simulink model "qcarLidarToGPS"  (R2021a)
settings: Solver=ode1  StartTime=0.0  StopTime=inf  FixedStep=1/15  RelTol=1e-3  EnableMultiTasking=on
undefined symbols (not defined in the file): qc_get_step_size
libraries: quarc_library x18, simulink x2
settings Model: SimulationMode=external  ExtModeTrigDuration=10000  Creator=PKaram  LastModifiedBy=mrushton
settings SolverCC: AlgebraicLoopSolver=TrustRegion  PositivePriorityOrder=on  AutoInsertRateTranBlk=on
settings DataIOCC: ReturnWorkspaceOutputs=off
settings DebuggingCC: ParameterPrecisionLossMsg=none  SFMachineParentedDataDiag=warning  ArithmeticOperatorsInVariantConditions=warning
settings HardwareCC: ProdBitPerLong=64  ProdLargestAtomicFloat=None  ProdEndianess=Unspecified  ProdHWDeviceType=Generic->64-bit Embedded Processor (LP64)
settings SFSimCC: SimUseLocalCustomCode=off  CustomCodeUndefinedFunction=UseInterfaceOnly
settings RTWCC: Description=QUARC Linux Nvidia Target (QCar) Using Toolchain  SystemTargetFile=quarc_linux_nvidia.tlc  TemplateMakefile=quarc_linux_nvidia_tmf  RTWUseLocalCustomCode=off  Toolchain=QUARC linux_nvidia | gmake (64-bit Windows)  BuildConfiguration=Faster Runs
settings CodeAppCC: StateflowObjectComments=on
settings STFCustomTargetCC: TargetLangStandard=C99 (ISO)  ConcurrentExecutionCompliant=on  SystemTargetFile=quarc_linux_nvidia.tlc
settings GRTTargetCC: ParMdlRefBuildCompliant=off  CompOptLevelCompliant=off  CombineOutputUpdateFcns=off  MatFileLogging=off  CPPClassGenCompliant=off  GRTInterface=on  ExtMode=on  ExtModeMexFile=quarc_comm  ExtModeMexArgs='-w -d /tmp -uri %u -pose_0 5.2,3.4,6.5','tcpip://192.168.55.1:17001'
settings ConfigComp: CovMetricSettings=dswe

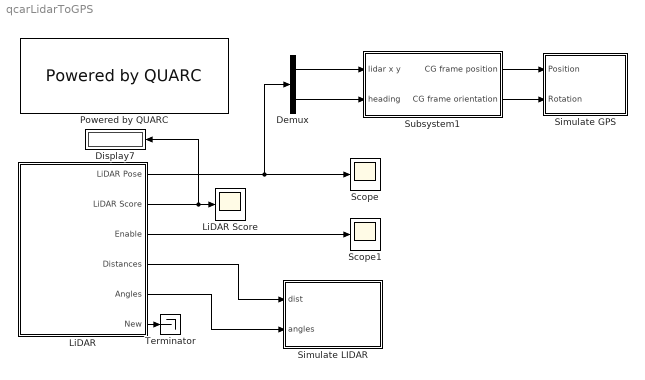
== system qcarLidarToGPS ==
  Demux : Demux  Outputs=[2 1]
  Display7 : Display
  LiDAR : Subsystem
  LiDAR Score : Scope
  Powered by QUARC : quarc_library/Logos/Powered by QUARC
  Scope : Scope
  Scope1 : Scope
  Simulate GPS : Subsystem
  Simulate LIDAR : Subsystem
  Subsystem1 : Subsystem
  Terminator : Terminator
  wires:
  LiDAR/2("LiDAR Score ") -> Display7/1, LiDAR Score/1
  LiDAR/3(Enable) -> Scope1/1
  LiDAR/1(LiDAR Pose) -> Scope/1, Demux/1
  Demux/1 -> Subsystem1/1(lidar x y)
  Subsystem1/1("CG frame position ") -> Simulate GPS/1(Position)
  Subsystem1/2(CG frame orientation) -> Simulate GPS/2(Rotation)
  Demux/2 -> Subsystem1/2(heading)
  LiDAR/4(Distances) -> Simulate LIDAR/1(dist)
  LiDAR/5(Angles) -> Simulate LIDAR/2(angles)
  LiDAR/6(New) -> Terminator/1

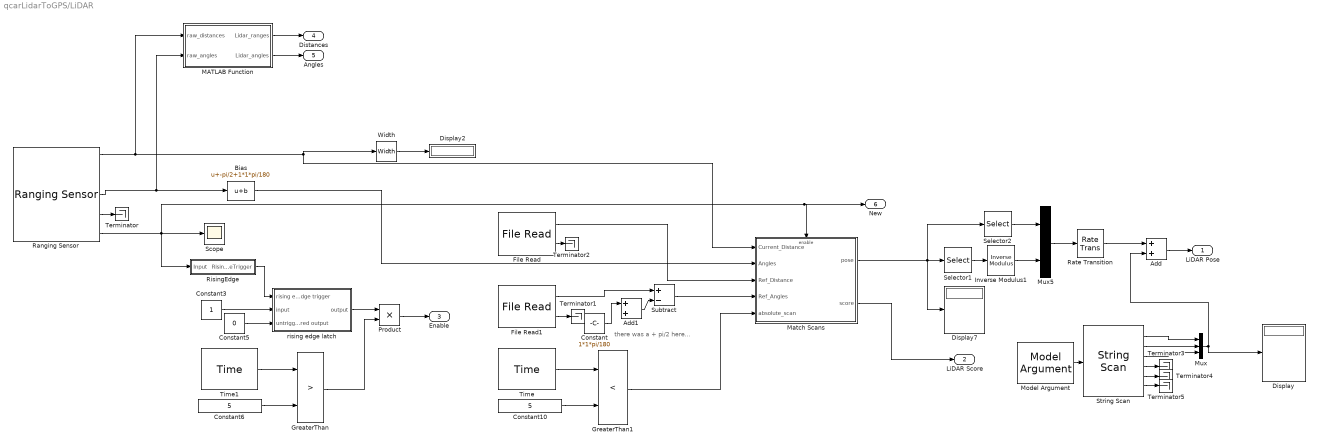
== system qcarLidarToGPS/LiDAR ==
  note: there was a + pi/2 here...
  Add : Sum
  Add1 : Sum
  Bias : Bias  Bias=-pi/2+1*1*pi/180
  Constant : Constant  Value=1*1*pi/180
  Constant10 : Constant  Value=5
  Constant3 : Constant
  Constant5 : Constant  Value=0
  Constant6 : Constant  Value=5
  Display : Display
  Display2 : Display
  Display7 : Display
  File Read : quarc_library/Sources/Signals/File Read  filename=distance_new.mat  format=MAT-file v.4  variable=distances  dimensions=[384, 1]  skip_lines=1  skip_columns=1  loop_count=0  sample_time=qc_get_step_size  data_type=double
      settings: AttributesFormatString=%<filename>  SourceProductName=QUARC Targets
  File Read1 : quarc_library/Sources/Signals/File Read  filename=angles_new.mat  format=MAT-file v.4  variable=angles  dimensions=[384, 1]  skip_lines=1  skip_columns=1  loop_count=0  sample_time=qc_get_step_size  data_type=double
      settings: AttributesFormatString=%<filename>  SourceProductName=QUARC Targets
  GreaterThan : RelationalOperator  Operator=>  OutDataTypeStr=boolean  RndMeth=Simplest
  GreaterThan1 : RelationalOperator  Operator=<  OutDataTypeStr=boolean  RndMeth=Simplest
  Inverse Modulus1 : quarc_library/Discontinuities/Inverse Modulus  modulus=2*pi  output_derivative=off  output_revolutions=off  max_x=Inf  min_x=-Inf
  MATLAB Function : MATLAB Function  TreatAsAtomicUnit=on
  Match Scans : Subsystem
  Model Argument : quarc_library/Sources/Signals/Model Argument  argument_name=pose_0  has_value=on  data_type_mode=Specify via dialog  data_type=char  max_length=80  default_value=0  variable_size=on
      settings: AttributesFormatString=(-%<argument_name>)  SourceProductName=QUARC Targets
  Mux : Mux  Inputs=3
  Mux5 : Mux  Inputs=2
  Product : Product
  Ranging Sensor : quarc_library/Devices/Third-Party/Sensors/Ranging Sensor  sensor_type=RPLidar LIDAR  uri=serial-cpu://localhost:2?baud='115200',word='8',parity='none',stop='1',flow='none',dsr='on'  ranging_distance=Long  timing_budget=0.033  measurement_period=0.040  output_mode=Variable-size output  samples_per_revolution=384  max_distance=0.050  max_angle=5  sample_time=qc_get_step_size  show_versions=off  active=on
      settings: SourceProductName=QUARC Targets
  Rate Transition : RateTransition
  RisingEdge : Subsystem
  Scope : Scope
  Selector1 : Selector  InputPortWidth=3  IndexOptions=Index vector (dialog)  Indices=3  OutputSizes=1
  Selector2 : Selector  InputPortWidth=3  IndexOptions=Index vector (dialog)  Indices=1:2  OutputSizes=1
  String Scan : quarc_library/Strings/String Scan  format_string=%e, %f, %g  max_length=80
      settings: SourceProductName=QUARC Targets
  Subtract : Sum  Inputs=+-
  Terminator{,1..5} (6 alike) : Terminator
  Time : quarc_library/Sources/Time/Time  time_source=Wall clock  sample_time=qc_get_step_size
  Time1 : quarc_library/Sources/Time/Time  time_source=Wall clock  sample_time=qc_get_step_size
  Width : Width
  rising edge latch : Subsystem
  LiDAR Pose : Outport
  "LiDAR Score " : Outport  Port=2
  Enable : Outport  Port=3
  Distances : Outport  Port=4
  Angles : Outport  Port=5
  New : Outport  Port=6
  wires:
  File Read/1 -> Match Scans/3(Ref_Distance)
  Width/1 -> Display2/1
  Ranging Sensor/1 -> MATLAB Function/1(raw_distances), Width/1, Match Scans/1(Current_Distance)
  Match Scans/1(pose) -> Display7/1, Selector2/1, Selector1/1
  Inverse Modulus1/1 -> Mux5/2
  Selector2/1 -> Mux5/1
  Selector1/1 -> Inverse Modulus1/1
  Constant6/1 -> GreaterThan/2
  RisingEdge/1(RisingEdgeTrigger) -> rising edge latch/1(rising edge trigger)
  Match Scans/2(score) -> "LiDAR Score "/1
  Product/1 -> Enable/1
  Constant3/1 -> rising edge latch/2(input)
  Constant5/1 -> rising edge latch/3(untriggered output)
  Constant10/1 -> GreaterThan1/2
  GreaterThan/1 -> Product/2
  Time/1 -> GreaterThan1/1
  GreaterThan1/1 -> Match Scans/5(absolute_scan)
  Time1/1 -> GreaterThan/1
  Ranging Sensor/3 -> MATLAB Function/2(raw_angles), Bias/1
  rising edge latch/1(output) -> Product/1
  Bias/1 -> Match Scans/2(Angles)
  Ranging Sensor/5 -> New/1, Match Scans/Enable, RisingEdge/1(Input), Scope/1
  File Read1/1 -> Subtract/1
  Subtract/1 -> Match Scans/4(Ref_Angles)
  Add/1 -> LiDAR Pose/1
  Rate Transition/1 -> Add/1
  Mux5/1 -> Rate Transition/1
  Ranging Sensor/4 -> Terminator/1
  File Read1/2 -> Terminator1/1
  File Read/2 -> Terminator2/1
  Model Argument/1 -> String Scan/1
  String Scan/3 -> Mux/3
  String Scan/2 -> Mux/2
  String Scan/1 -> Mux/1
  Mux/1 -> Display/1, Add/2
  String Scan/4 -> Terminator3/1
  String Scan/5 -> Terminator4/1
  String Scan/6 -> Terminator5/1
  Add1/1 -> Subtract/2
  Constant/1 -> Add1/1
  MATLAB Function/1(Lidar_ranges) -> Distances/1
  MATLAB Function/2(Lidar_angles) -> Angles/1

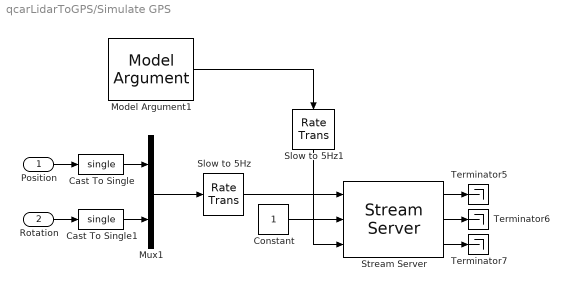
== system qcarLidarToGPS/Simulate GPS ==
  Position : Inport
  Rotation : Inport  Port=2
  Cast To Single : DataTypeConversion  OutDataTypeStr=single
  Cast To Single1 : DataTypeConversion  OutDataTypeStr=single
  Constant : Constant
  Model Argument1 : quarc_library/Sources/Signals/Model Argument  argument_name=uri_gps  has_value=on  data_type_mode=Specify via dialog  data_type=char  max_length=80  default_value=0  default_string=tcpip://remotehost:18967  variable_size=off
      settings: AttributesFormatString=(-%<argument_name>)  SourceProductName=QUARC Targets
  Mux1 : Mux  Inputs=2
  Slow to 5Hz : RateTransition  OutPortSampleTime=qc_get_step_size*3
  Slow to 5Hz1 : RateTransition  OutPortSampleTime=qc_get_step_size*3
  Stream Server : quarc_library/Communications/Basic/Stream Server  uri_source=External input port  uri=tcpip://remotehost:18967  send_buffer_size=6*4  receive_buffer_size=1  byte_order=little endian (Intel - LSB first)  optimization=Minimum latency  send_options=Send most recent data  receive_options=Do not receive data  default_value=[0]  sample_time=qc_get_step_size*3  active=off  implementation=Use blocking I/O in a separate thread  send_fifo_size=1000  receive_fifo_size=1000  send_priority=0  receive_priority=0  send_dimensions=off  receive_dimensions=off  max_dimensions=-1  data_type=Inherited via back propagation  type_expr=BusObject
  Terminator5 : Terminator
  Terminator6 : Terminator
  Terminator7 : Terminator
  wires:
  Rotation/1 -> Cast To Single1/1
  Stream Server/1 -> Terminator5/1
  Stream Server/2 -> Terminator6/1
  Stream Server/3 -> Terminator7/1
  Constant/1 -> Stream Server/2
  Position/1 -> Cast To Single/1
  Mux1/1 -> Slow to 5Hz/1
  Slow to 5Hz/1 -> Stream Server/1
  Model Argument1/1 -> Slow to 5Hz1/1
  Slow to 5Hz1/1 -> Stream Server/3
  Cast To Single/1 -> Mux1/1
  Cast To Single1/1 -> Mux1/2

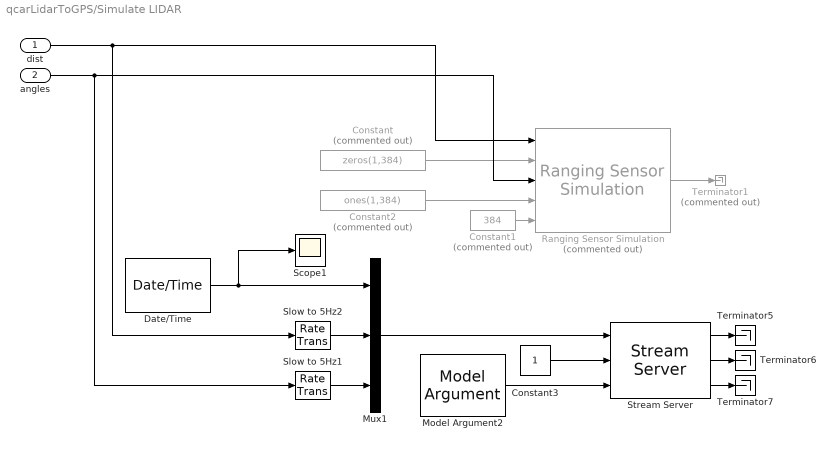
== system qcarLidarToGPS/Simulate LIDAR ==
  dist : Inport
  angles : Inport  Port=2
  Constant : Constant  Commented=on  Value=zeros(1,384)
  Constant1 : Constant  Commented=on  Value=384
  Constant2 : Constant  Commented=on  Value=ones(1,384)
  Constant3 : Constant
  Date/Time : quarc_library/Sources/Time/Date//Time  show_date=off  show_time=off  show_epoch=on  use_utc=off  sample_time=qc_get_step_size*3
      settings: SourceProductName=QUARC Targets
  Model Argument2 : quarc_library/Sources/Signals/Model Argument  argument_name=uri_gps  has_value=on  data_type_mode=Specify via dialog  data_type=char  max_length=80  default_value=0  default_string=tcpip://remotehost:18968  variable_size=off
      settings: AttributesFormatString=(-%<argument_name>)  SourceProductName=QUARC Targets
  Mux1 : Mux  Inputs=3
  Ranging Sensor Simulation : quarc_library/Devices/Third-Party/Sensors/Ranging Sensor Simulation  Commented=on  sensor_type=RPLIDAR A2  uri_source=Specify via dialog (do not evaluate)  uri=tcpip://localhost:18966  sample_time=qc_get_step_size  show_in_use=off  variable_size=off  active=on
      settings: AttributesFormatString="\"tcpip://localhost:18966\""  SourceProductName=QUARC Targets
  Scope1 : Scope
  Slow to 5Hz1 : RateTransition  OutPortSampleTime=qc_get_step_size*3
  Slow to 5Hz2 : RateTransition  OutPortSampleTime=qc_get_step_size*3
  Stream Server : quarc_library/Communications/Basic/Stream Server  uri_source=External input port  uri=tcpip://remotehost:18967  send_buffer_size=(1 + 2*384) * 8  receive_buffer_size=1  byte_order=little endian (Intel - LSB first)  optimization=Minimum latency  send_options=Send most recent data  receive_options=Do not receive data  default_value=[0]  sample_time=qc_get_step_size*3  active=off  implementation=Use non-blocking I/O  send_fifo_size=2  receive_fifo_size=1000  send_priority=0  receive_priority=0  send_dimensions=off  receive_dimensions=off  max_dimensions=-1  data_type=Inherited via back propagation  type_expr=BusObject
  Terminator1 : Terminator  Commented=on
  Terminator5 : Terminator
  Terminator6 : Terminator
  Terminator7 : Terminator
  wires:
  Constant/1 -> Ranging Sensor Simulation/2
  Constant1/1 -> Ranging Sensor Simulation/5
  Constant2/1 -> Ranging Sensor Simulation/4
  Ranging Sensor Simulation/1 -> Terminator1/1
  Model Argument2/1 -> Stream Server/3
  Constant3/1 -> Stream Server/2
  Stream Server/1 -> Terminator5/1
  Stream Server/3 -> Terminator7/1
  Stream Server/2 -> Terminator6/1
  Mux1/1 -> Stream Server/1
  Date/Time/1 -> Mux1/1, Scope1/1
  Slow to 5Hz1/1 -> Mux1/3
  Slow to 5Hz2/1 -> Mux1/2
  dist/1 -> Slow to 5Hz2/1, Ranging Sensor Simulation/1
  angles/1 -> Slow to 5Hz1/1, Ranging Sensor Simulation/3

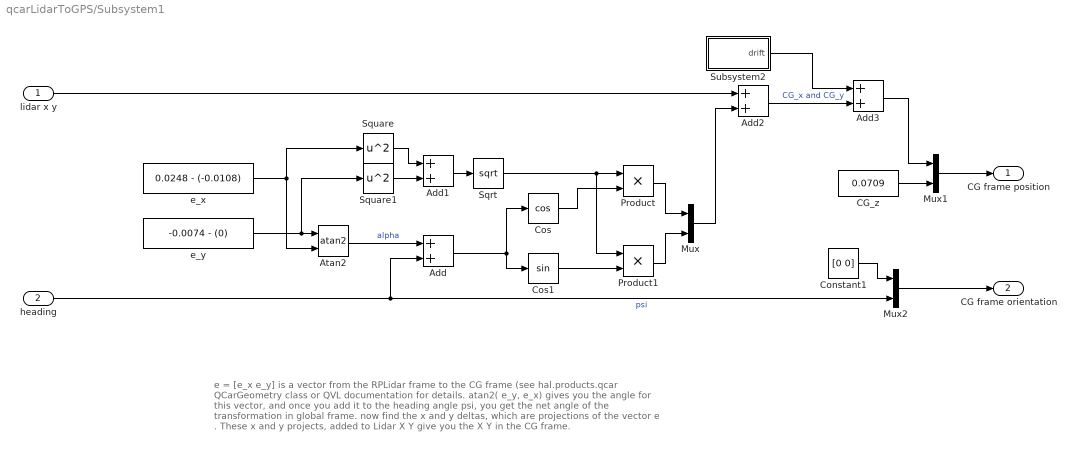
== system qcarLidarToGPS/Subsystem1 ==
  note: e = [e_x e_y] is a vector from the RPLidar frame to the CG frame (see hal.products.qcar QCarGeometry class or QVL documentation for details.
      |
      | atan2( e_y, e_x) gives you the angle for this vector, and once you add it to the heading angle psi, you get the net angle of the transformation in global frame. now find the x and y deltas, which are projections of the vector e . These x and y projects, added to Lidar X Y give you the X Y in the CG frame.
  lidar x y : Inport
  heading : Inport  Port=2
  Add{,1..3} (4 alike) : Sum
  Atan2 : Trigonometry  Operator=atan2
  CG_z : Constant  Value=0.0709
  Constant1 : Constant  Value=[0 0]
  Cos : Trigonometry  Operator=cos
  Cos1 : Trigonometry
  Mux : Mux  Inputs=2
  Mux1 : Mux  Inputs=2
  Mux2 : Mux  Inputs=2
  Product : Product
  Product1 : Product
  Sqrt : Sqrt  SaturateOnIntegerOverflow=on
  Square : Math  Operator=square  SaturateOnIntegerOverflow=on
  Square1 : Math  Operator=square  SaturateOnIntegerOverflow=on
  Subsystem2 : Subsystem
  e_x : Constant  Value=0.0248 - (-0.0108)
  e_y : Constant  Value=-0.0074 - (0)
  "CG frame position " : Outport
  CG frame orientation : Outport  Port=2
  wires:
  e_y/1 -> Square1/1, Atan2/1
  e_x/1 -> Square/1, Atan2/2
  Atan2/1 -> Add/1  "alpha"
  heading/1 -> Mux2/2, Add/2  "psi"
  Square/1 -> Add1/1
  Square1/1 -> Add1/2
  Add1/1 -> Sqrt/1
  Add/1 -> Cos1/1, Cos/1
  Sqrt/1 -> Product1/1, Product/1
  Cos/1 -> Product/2
  Cos1/1 -> Product1/2
  Product/1 -> Mux/1
  Product1/1 -> Mux/2
  Mux/1 -> Add2/2
  lidar x y/1 -> Add2/1
  Add2/1 -> Add3/2  "CG_x and CG_y"
  CG_z/1 -> Mux1/2
  Constant1/1 -> Mux2/1
  Mux1/1 -> "CG frame position "/1
  Mux2/1 -> CG frame orientation/1
  Subsystem2/1(drift) -> Add3/1
  Add3/1 -> Mux1/1

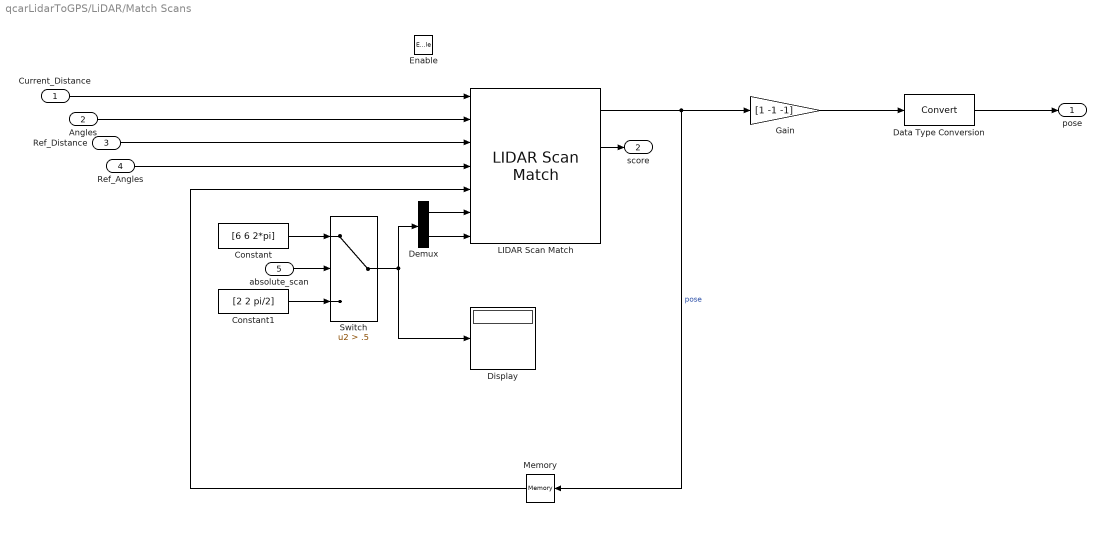
== system qcarLidarToGPS/LiDAR/Match Scans ==
  Current_Distance : Inport
  Angles : Inport  Port=2
  Ref_Distance : Inport  Port=3
  Ref_Angles : Inport  Port=4
  absolute_scan : Inport  Port=5
  Enable : EnablePort
  Constant : Constant  Value=[6 6 2*pi]
  Constant1 : Constant  Value=[2 2 pi/2]
  Data Type Conversion : DataTypeConversion
  Demux : Demux  Outputs=2
  Display : Display
  Gain : Gain  Gain=[1 -1 -1]
  LIDAR Scan Match : quarc_library/Image Processing/Generic/LIDAR Scan Match  mode=Variable-size input  resolution=30  max_range=6  use_initial_pose=on
      settings: SourceProductName=QUARC Targets
  Memory : Memory  InitialCondition=[0 0 0]  InheritSampleTime=on  LinearizeMemory=on  LinearizeAsDelay=on
  Switch : Switch  Criteria=u2 > Threshold  Threshold=.5
  pose : Outport
  score : Outport  Port=2
  wires:
  LIDAR Scan Match/1 -> Memory/1, Gain/1  "pose"
  Current_Distance/1 -> LIDAR Scan Match/1
  Ref_Distance/1 -> LIDAR Scan Match/3
  Angles/1 -> LIDAR Scan Match/2
  Ref_Angles/1 -> LIDAR Scan Match/4
  Gain/1 -> Data Type Conversion/1
  LIDAR Scan Match/2 -> score/1
  Memory/1 -> LIDAR Scan Match/5
  absolute_scan/1 -> Switch/2
  Switch/1 -> Demux/1, Display/1
  Demux/1 -> LIDAR Scan Match/6
  Demux/2 -> LIDAR Scan Match/7
  Constant/1 -> Switch/1
  Constant1/1 -> Switch/3
  Data Type Conversion/1 -> pose/1

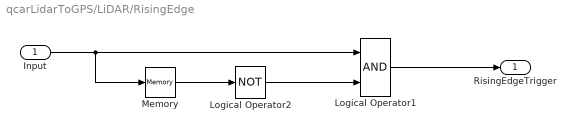
== system qcarLidarToGPS/LiDAR/RisingEdge ==
  Input : Inport
  Logical Operator1 : Logic  AllPortsSameDT=off
  Logical Operator2 : Logic  Operator=NOT  AllPortsSameDT=off
  Memory : Memory  InheritSampleTime=on  LinearizeMemory=on
  RisingEdgeTrigger : Outport  VectorParamsAs1DForOutWhenUnconnected=off
  wires:
  Logical Operator1/1 -> RisingEdgeTrigger/1
  Logical Operator2/1 -> Logical Operator1/2
  Memory/1 -> Logical Operator2/1
  Input/1 -> Logical Operator1/1, Memory/1

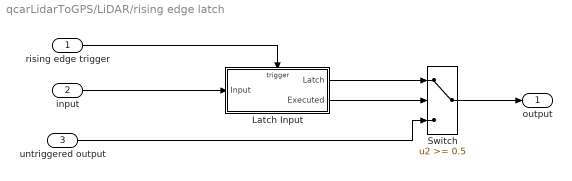
== system qcarLidarToGPS/LiDAR/rising edge latch ==
  rising edge trigger : Inport
  input : Inport  Port=2
  untriggered output : Inport  Port=3
  Latch Input : Subsystem  TreatAsAtomicUnit=on
  Switch : Switch  Threshold=0.5
  output : Outport  VectorParamsAs1DForOutWhenUnconnected=off
  wires:
  untriggered output/1 -> Switch/3
  Switch/1 -> output/1
  Latch Input/1(Latch) -> Switch/1
  Latch Input/2(Executed) -> Switch/2
  input/1 -> Latch Input/1(Input)
  rising edge trigger/1 -> Latch Input/Trigger

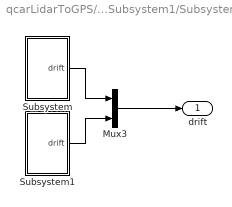
== system qcarLidarToGPS/Subsystem1/Subsystem2 ==
  Mux3 : Mux  Inputs=2
  Subsystem : Subsystem
  Subsystem1 : Subsystem
  drift : Outport
  wires:
  Subsystem1/1(drift) -> Mux3/2
  Subsystem/1(drift) -> Mux3/1
  Mux3/1 -> drift/1

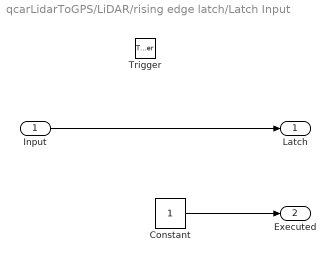
== system qcarLidarToGPS/LiDAR/rising edge latch/Latch Input ==
  Input : Inport
  Trigger : TriggerPort  VariantControl=(inherit)
  Constant : Constant
  Latch : Outport  VectorParamsAs1DForOutWhenUnconnected=off
  Executed : Outport  Port=2  VectorParamsAs1DForOutWhenUnconnected=off
  wires:
  Constant/1 -> Executed/1
  Input/1 -> Latch/1

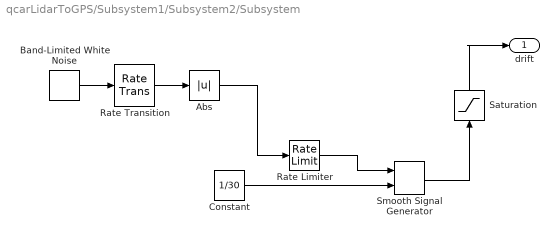
== system qcarLidarToGPS/Subsystem1/Subsystem2/Subsystem ==
  Abs : Abs
  Band-Limited White Noise : simulink/Sources/Band-Limited White Noise  Cov=[0.002]  Ts=5  seed=randi(23341)
  Constant : Constant  Value=1/30  SampleTime=1/15
  Rate Limiter : RateLimiter  RisingSlewLimit=0.1  SampleTimeMode=inherited
  Rate Transition : RateTransition
  Saturation : Saturate  UpperLimit=0.07/sqrt(2)  LowerLimit=-0.07/sqrt(2)
  Smooth Signal Generator : quarc_library/Sources/Signals/Smooth Signal Generator  signal_type=Sine  source=External (input ports)  amplitude=1  frequency=1  initial_phase=randi(360)*pi/180  sample_time=qc_get_step_size  output_cos=off
      settings: SourceProductName=QUARC Targets
  drift : Outport
  wires:
  Band-Limited White Noise/1 -> Rate Transition/1
  Smooth Signal Generator/1 -> Saturation/1
  Abs/1 -> Rate Limiter/1
  Rate Limiter/1 -> Smooth Signal Generator/1
  Rate Transition/1 -> Abs/1
  Constant/1 -> Smooth Signal Generator/2
  Saturation/1 -> drift/1

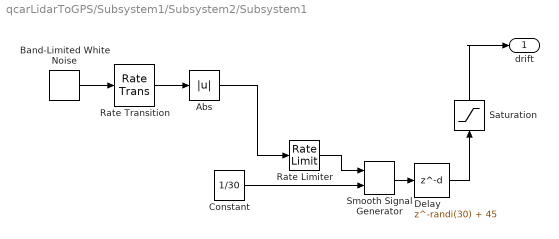
== system qcarLidarToGPS/Subsystem1/Subsystem2/Subsystem1 ==
  Abs : Abs
  Band-Limited White Noise : simulink/Sources/Band-Limited White Noise  Cov=[0.002]  Ts=5  seed=randi(23341)
  Constant : Constant  Value=1/30  SampleTime=1/15
  Delay : Delay  DelayLength=randi(30) + 45
  Rate Limiter : RateLimiter  RisingSlewLimit=0.1  SampleTimeMode=inherited
  Rate Transition : RateTransition
  Saturation : Saturate  UpperLimit=0.07/sqrt(2)  LowerLimit=-0.07/sqrt(2)
  Smooth Signal Generator : quarc_library/Sources/Signals/Smooth Signal Generator  signal_type=Sine  source=External (input ports)  amplitude=1  frequency=1  initial_phase=randi(360)*pi/180  sample_time=qc_get_step_size  output_cos=off
      settings: SourceProductName=QUARC Targets
  drift : Outport
  wires:
  Constant/1 -> Smooth Signal Generator/2
  Rate Transition/1 -> Abs/1
  Rate Limiter/1 -> Smooth Signal Generator/1
  Abs/1 -> Rate Limiter/1
  Smooth Signal Generator/1 -> Delay/1
  Band-Limited White Noise/1 -> Rate Transition/1
  Saturation/1 -> drift/1
  Delay/1 -> Saturation/1

== matlab function qcarLidarToGPS/LiDAR/MATLAB Function ==
  data: raw_distances input size=384; Lidar_ranges output; raw_angles input size=384; Lidar_angles output
function [Lidar_ranges,Lidar_angles]= fcn(raw_distances, raw_angles)

%  Fixed sized vector used for streaming the LiDAR values 
Lidar_ranges = zeros(384,1);
Lidar_angles = zeros(384,1);


Lidar_ranges(:)  = raw_distances;
Lidar_angles (:) =  raw_angles;
